simulink model "V_Hz_control_sim"  (R2023a)
settings: Solver=VariableStepAuto  StartTime=0.0  StopTime=100  RelTol=1e-3
values from neighbouring files (symbols this model uses):
  B = 0.068    [V_Hz_control.m]
  I = 0.4    [V_Hz_control.m]
  K = 1:500    [V_Hz_control.m]
  kiw = 0.68*100    (= 68)    [V_Hz_control.m]
  kpw = 4*100    (= 400)    [V_Hz_control.m]
  Lks = Ls- Lm^2/Lr    (= 0.00442538071066)    [V_Hz_control.m]
  Lm = 57e-3    (= 0.057)    [V_Hz_control.m]
  np = 3    [V_Hz_control.m]
  Rr = 0.175    [V_Hz_control.m]
  Rs = 0.24    [V_Hz_control.m]
undefined symbols (not defined in the file or in its folder): j
libraries: slpidlib x1
settings Model: Creator=Andrea  LastModifiedBy=Andrea

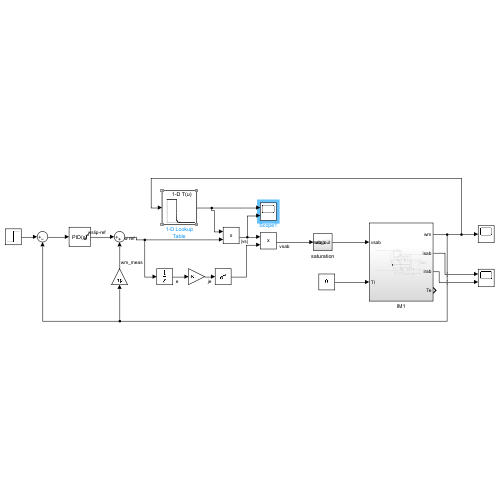
[thumbnail: Simulink's stored preview of the top-level diagram]
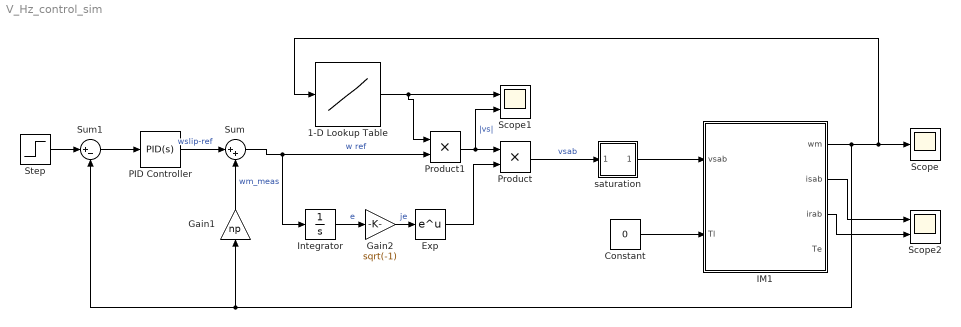
== system V_Hz_control_sim ==
  1-D Lookup Table : Lookup_n-D  NumberOfTableDimensions=1  BreakpointsForDimension1=[1:500]  Table=K  InternalRulePriority=Speed  RndMeth=Simplest
  Constant : Constant  Value=0
  Exp : Math
  Gain1 : Gain  Gain=np
  Gain2 : Gain  Gain=sqrt(-1)
  IM1 : Subsystem
  Integrator : Integrator
  PID Controller : slpidlib/PID Controller  Controller=PID  Form=Parallel  TimeDomain=Continuous-time  UseExternalTs=off  SampleTime=-1  IntegratorMethod=Forward Euler  FilterMethod=Forward Euler  ControllerParametersSource=internal  P=kpw  I=kiw  UseKiTs=off  D=0  N=100  UseFilter=on  TunerSelectOption=Transfer Function Based (PID Tuner App)  InitialConditionSource=internal  InitialConditionForIntegrator=0  InitialConditionForFilter=0  DifferentiatorICPrevScaledInput=0  ExternalReset=none  TrackingMode=off  Kt=1  LimitOutput=on  SatLimitsSource=internal  UpperSaturationLimit=0.7  LowerSaturationLimit=0  LinearizeAsGain=on  AntiWindupMode=back-calculation  Kb=kiw/kpw  LimitIntegrator=off  UpperIntegratorSaturationLimit=inf  LowerIntegratorSaturationLimit=-inf  POutMin=[]  POutMax=[]  IOutMin=[]  IOutMax=[]  DOutMin=[]  DOutMax=[]  NOutMin=[]  NOutMax=[]  SumOutMin=[]  SumOutMax=[]  SaturationOutMin=[]  SaturationOutMax=[]  PParamMin=[]  PParamMax=[]  IParamMin=[]  IParamMax=[]  DParamMin=[]  DParamMax=[]  NParamMin=[]  NParamMax=[]  KbParamMin=[]  KbParamMax=[]  KtParamMin=[]  KtParamMax=[]  KbOutMin=[]  KbOutMax=[]  KtOutMin=[]  KtOutMax=[]  IntegratorOutMin=[]  IntegratorOutMax=[]  FilterOutMin=[]  FilterOutMax=[]  SumI1OutMin=[]  SumI1OutMax=[]  SumI2OutMin=[]  SumI2OutMax=[]  SumI3OutMin=[]  SumI3OutMax=[]  SumI4OutMin=[]  SumI4OutMax=[]  SumDOutMin=[]  SumDOutMax=[]  DifferentiatorOutMin=[]  DifferentiatorOutMax=[]  FilterDiffOutCoefMin=[]  FilterDiffOutCoefMax=[]  ReciprocalOutMin=[]  ReciprocalOutMax=[]  SumDenOutMin=[]  SumDenOutMax=[]  SumNumOutMin=[]  SumNumOutMax=[]  DivideOutMin=[]  DivideOutMax=[]  UdiffTsProdOutMin=[]  UdiffTsProdOutMax=[]  NTsProdOutMin=[]  NTsProdOutMax=[]  UintegralTsProdOutMin=[]  UintegralTsProdOutMax=[]  UngainTsProdOutMin=[]  UngainTsProdOutMax=[]  ClampingZeroOutDataTypeStr=Inherit: Inherit via back propagation  ClampingZeroOutMin=[]  ClampingZeroOutMax=[]  FilterDenConstantOutDataTypeStr=Inherit: Inherit via back propagation  FilterDenConstantOutMin=[]  FilterDenConstantOutMax=[]  PCopyOutDataTypeStr=Inherit: Inherit via back propagation  PCopyOutMin=[]  PCopyOutMax=[]  NCopyOutDataTypeStr=Inherit: Inherit via back propagation  NCopyOutMin=[]  NCopyOutMax=[]  IntegratorContinuousStateAttributes=''  IntegratorStateMustResolveToSignalObject=off  IntegratorRTWStateStorageClass=Auto  FilterContinuousStateAttributes=''  FilterStateMustResolveToSignalObject=off  FilterRTWStateStorageClass=Auto  ParallelPVariant=InternalParameters  IdealPVariant=Disabled  IVariant=InternalParameters  DVariant=InternalParameters  IntegratorVariant=Continuous  SatVariant=Enabled  AWVariant=BackCalculation  PCopyVariant=Disabled  TRVariant=Disabled  FdbkBlocksVariant=Forward  IdealPFdbkVariant=Disabled  SatFdbkVariant=Disabled  DerivativeFilterVariant=ContFilter  NVariant=InternalParameters  NCopyVariant=Disabled  FilterICVariant=InternalICsFilter  IntegratorICVariant=InternalICs  ExternalResetVariant=Disabled  TRSumVariant=Passthrough  SumFdbkVariant=Disabled  SumVariant=Sum_PID  TsampFilterVariant=InternalTs  TsampNgainVariant=Passthrough  TsampIntegralVariant=Disabled_SignalSpec  ExternalSaturationOutDataTypeStr=Inherit: Same as second input
  Product : Product
  Product1 : Product
  Scope : Scope
  Scope1 : Scope  NumInputPorts=2
  Scope2 : Scope  NumInputPorts=2
  Step : Step  After=300  SampleTime=0
  Sum : Sum  Inputs=|++
  Sum1 : Sum  Inputs=|+-
  saturation : Subsystem
  wires:
  Integrator/1 -> Gain2/1  "e"
  Exp/1 -> Product/2
  Gain2/1 -> Exp/1  "je"
  IM1/1(wm) -> Sum1/2, Gain1/1, 1-D Lookup Table/1, Scope/1
  IM1/3(irab) -> Scope2/2
  IM1/2(isab) -> Scope2/1
  Constant/1 -> IM1/2(Tl)
  Step/1 -> Sum1/1
  Product/1 -> saturation/1(vsab)  "vsab"
  saturation/1(vsab_out) -> IM1/1(vsab)
  Product1/1 -> Scope1/2, Product/1  "|vs|"
  PID Controller/1 -> Sum/1  "wslip-ref"
  Gain1/1 -> Sum/2  "wm_meas"
  Sum/1 -> Integrator/1, Product1/2  "w ref"
  Sum1/1 -> PID Controller/1
  1-D Lookup Table/1 -> Product1/1, Scope1/1

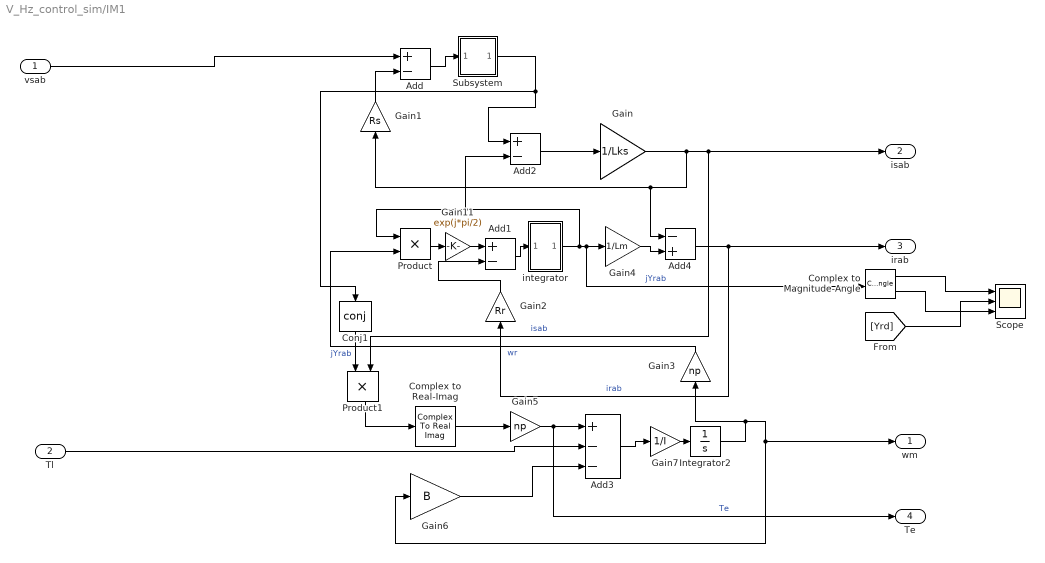
== system V_Hz_control_sim/IM1 ==
  vsab : Inport
  Tl : Inport  Port=2
  Add : Sum  Inputs=+-
  Add1 : Sum  Inputs=+-
  Add2 : Sum  Inputs=+-
  Add3 : Sum  Inputs=+--
  Add4 : Sum  Inputs=-+
  Complex to Magnitude-Angle : ComplexToMagnitudeAngle
  Complex to Real-Imag : ComplexToRealImag  Output=Imag
  Conj1 : Math  Operator=conj
  Gain : Gain  Gain=1/Lks
  Gain1 : Gain  Gain=Rs
  Gain11 : Gain  Gain=exp(j*pi/2)
  Gain2 : Gain  Gain=Rr
  Gain3 : Gain  Gain=np
  Gain4 : Gain  Gain=1/Lm
  Gain5 : Gain  Gain=np
  Gain6 : Gain  Gain=B
  Gain7 : Gain  Gain=1/I
  Integrator2 : Integrator
  Product : Product
  Product1 : Product
  Scope : Scope  NumInputPorts=3
  Subsystem : Subsystem
  integrator : Subsystem
  wm : Outport
  isab : Outport  Port=2
      settings: SignalType=complex
  irab : Outport  Port=3
      settings: SignalType=complex
  Te : Outport  Port=4
  wires:
  Add2/1 -> Gain/1
  Add4/1 -> Gain2/1, irab/1  "irab"
  Gain/1 -> Add4/1, Gain1/1, Product1/2, isab/1  "isab"
  Gain6/1 -> Add3/3
  Gain4/1 -> Add4/2
  Gain1/1 -> Add/2
  Gain5/1 -> Add3/1, Te/1  "Te"
  Product1/1 -> Complex to Real-Imag/1
  Conj1/1 -> Product1/1  "jYrab"
  Complex to Real-Imag/1 -> Gain5/1
  Gain2/1 -> Add1/2
  Add3/1 -> Gain7/1
  Gain7/1 -> Integrator2/1
  Gain3/1 -> Product/2  "wr"
  vsab/1 -> Add/1
  Tl/1 -> Add3/2
  Integrator2/1 -> wm/1, Gain6/1, Gain3/1
  Add1/1 -> integrator/1(In1)
  Subsystem/1(Ysab) -> Add2/1, Conj1/1
  Add/1 -> Subsystem/1(In1)
  Gain11/1 -> Add1/1
  Product/1 -> Gain11/1
  Complex to Magnitude-Angle/2 -> Scope/3
  [Yrd] -> Scope/2
  integrator/1(Yrab) -> Product/1, Add2/2, Complex to Magnitude-Angle/1, Gain4/1  "jYrab"
  Complex to Magnitude-Angle/1 -> Scope/1

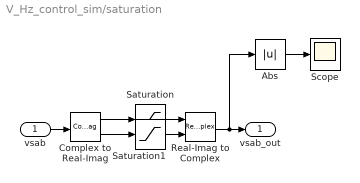
== system V_Hz_control_sim/saturation ==
  vsab : Inport
  Abs : Abs  SaturateOnIntegerOverflow=off
  Complex to Real-Imag : ComplexToRealImag
  Real-Imag to Complex : RealImagToComplex
  Saturation : Saturate  UpperLimit=380*sqrt(3/2)  LowerLimit=-380*sqrt(3/2)
  Saturation1 : Saturate  UpperLimit=380*sqrt(3/2)  LowerLimit=-380*sqrt(3/2)
  Scope : Scope
  vsab_out : Outport
  wires:
  Saturation1/1 -> Real-Imag to Complex/2
  Complex to Real-Imag/2 -> Saturation1/1
  Complex to Real-Imag/1 -> Saturation/1
  Saturation/1 -> Real-Imag to Complex/1
  vsab/1 -> Complex to Real-Imag/1
  Real-Imag to Complex/1 -> Abs/1, vsab_out/1
  Abs/1 -> Scope/1

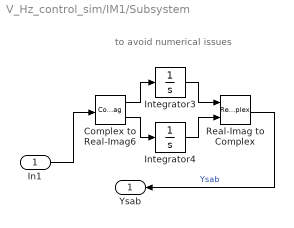
== system V_Hz_control_sim/IM1/Subsystem ==
  note: to avoid numerical issues
  In1 : Inport
  Complex to Real-Imag6 : ComplexToRealImag
  Integrator3 : Integrator
  Integrator4 : Integrator
  Real-Imag to Complex : RealImagToComplex
  Ysab : Outport
  wires:
  In1/1 -> Complex to Real-Imag6/1
  Complex to Real-Imag6/2 -> Integrator4/1
  Complex to Real-Imag6/1 -> Integrator3/1
  Integrator3/1 -> Real-Imag to Complex/1
  Real-Imag to Complex/1 -> Ysab/1  "Ysab"
  Integrator4/1 -> Real-Imag to Complex/2

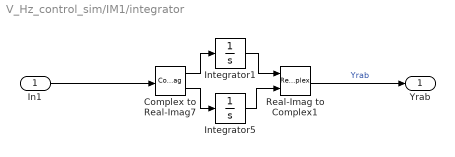
== system V_Hz_control_sim/IM1/integrator ==
  In1 : Inport
  Complex to Real-Imag7 : ComplexToRealImag
  Integrator1 : Integrator
  Integrator5 : Integrator
  Real-Imag to Complex1 : RealImagToComplex
  Yrab : Outport
  wires:
  Complex to Real-Imag7/2 -> Integrator5/1
  Integrator1/1 -> Real-Imag to Complex1/1
  Real-Imag to Complex1/1 -> Yrab/1  "Yrab"
  Integrator5/1 -> Real-Imag to Complex1/2
  Complex to Real-Imag7/1 -> Integrator1/1
  In1/1 -> Complex to Real-Imag7/1
